simulink model "Observer_Model"  (R2023b)
settings: Solver=VariableStepAuto  StartTime=0.0  StopTime=10.0  RelTol=1e-3
values from neighbouring files (symbols this model uses):
  A = [0 1; -w_n^2 -2*zeta*w_n]    [Lab_2_Prep.m]    (also in UnderDampedFitTest.m)
  B = [0; 1]    [Lab_2_Prep.m]    (also in UnderDampedFitTest.m)
  C = [1, 0]    [Lab_2_Prep.m]    (also in UnderDampedFitTest.m)
  D = 0    [Lab_2_Prep.m]    (also in UnderDampedFitTest.m)
  K = acker(A,B,poles)    [Lab_2_Prep.m]    (also in UnderDampedFitTest.m)
  L = acker(A',C',Pl)'    [Lab_2_Prep.m]    (also in UnderDampedFitTest.m)
  V = -1/(C*inv(A-B*K)*B)    [Lab_2_Prep.m]    (also in UnderDampedFitTest.m)
libraries: mci_models x1
settings Model: Creator=jojos  LastModifiedBy=jojos

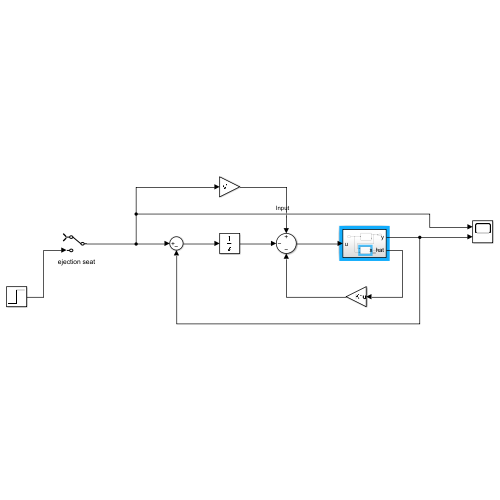
[thumbnail: Simulink's stored preview of the top-level diagram]
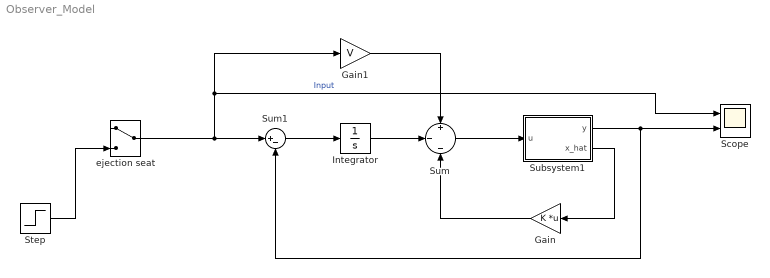
== system Observer_Model ==
  Gain : Gain  Gain=K  Multiplication=Matrix(K*u)
  Gain1 : Gain  Gain=V
  Integrator : Integrator
  Scope : Scope  NumInputPorts=2
  Step : Step  SampleTime=0
  Subsystem1 : Subsystem
  Sum : Sum  Inputs=+|-|-
  Sum1 : Sum  Inputs=|+-
  ejection seat : ManualSwitch
  wires:
  Sum/1 -> Subsystem1/1(u)
  Subsystem1/2(x_hat) -> Gain/1
  Gain/1 -> Sum/3
  Sum1/1 -> Integrator/1
  Integrator/1 -> Sum/2
  Subsystem1/1(y) -> Scope/2, Sum1/2
  ejection seat/1 -> Gain1/1, Scope/1, Sum1/1  "Input"
  Gain1/1 -> Sum/1
  Step/1 -> ejection seat/2

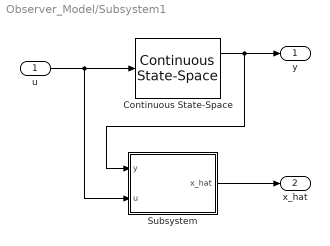
== system Observer_Model/Subsystem1 ==
  u : Inport
  Continuous State-Space : mci_models/State-Space Blocks/Continuous State-Space  A=A  B=B  C=C  D=D  x0=x_init
      settings: SourceProductName=MCI Models
  Subsystem : Subsystem
  y : Outport
  x_hat : Outport  Port=2
  wires:
  Subsystem/1(x_hat) -> x_hat/1
  Continuous State-Space/1 -> Subsystem/1(y), y/1
  u/1 -> Subsystem/2(u), Continuous State-Space/1

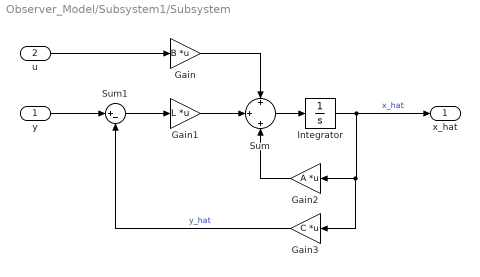
== system Observer_Model/Subsystem1/Subsystem ==
  y : Inport
  u : Inport  Port=2
  Gain : Gain  Gain=B  Multiplication=Matrix(K*u)
  Gain1 : Gain  Gain=L  Multiplication=Matrix(K*u)
  Gain2 : Gain  Gain=A  Multiplication=Matrix(K*u)
  Gain3 : Gain  Gain=C  Multiplication=Matrix(K*u)
  Integrator : Integrator
  Sum : Sum  Inputs=+|+|+
  Sum1 : Sum  Inputs=|+-
  x_hat : Outport
  wires:
  Integrator/1 -> x_hat/1, Gain3/1, Gain2/1  "x_hat"
  Gain2/1 -> Sum/3
  Sum1/1 -> Gain1/1
  Gain1/1 -> Sum/2
  Gain/1 -> Sum/1
  Gain3/1 -> Sum1/2  "y_hat"
  Sum/1 -> Integrator/1
  y/1 -> Sum1/1
  u/1 -> Gain/1
